simulink subsystem "anode_subsystem_basic_hctrl"  (R2023a)
settings: Solver=VariableStepAuto  StartTime=0.0  StopTime=10.0  RelTol=1e-3
values from neighbouring files (symbols this model uses):
  densityHydrogen = 0.0899    [All_Properties.mat]    (also in Valve_Init.m; anode_subsystem_parameters.m)
  Kv_VL6112 = 0.8    [All_Properties.mat]    (also in anode_subsystem_parameters.m)
undefined symbols (not defined in the file or in its folder): init_Parameters, ts
libraries: simulink x2, eeGeneralControl x1, slpidlib x1
settings Model: Creator=stefan.notter  LastModifiedBy=stefan.notter

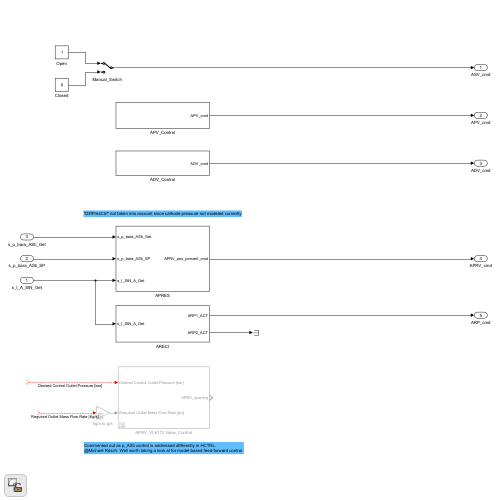
[thumbnail: Simulink's stored preview of the top-level diagram]
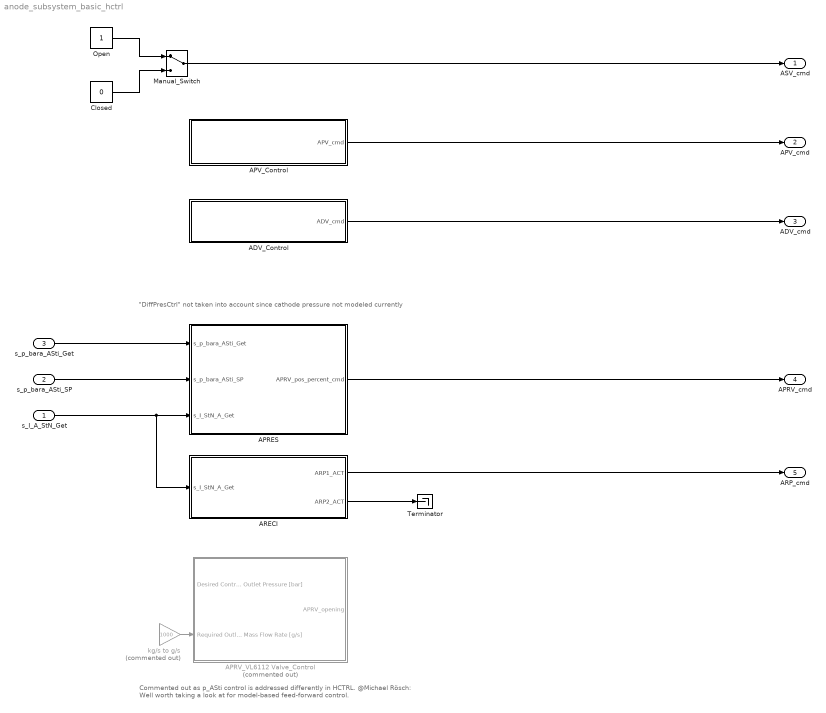
== system anode_subsystem_basic_hctrl ==
  note: Commented out as p_ASti control is addressed differently in HCTRL.
      | @Michael Rösch: Well worth taking a look at for model-based feed-forward control.
  note: "DiffPresCtrl" not taken into account since cathode pressure not modeled currently
  s_I_A_StN_Get : Inport
  s_p_bara_ASti_SP : Inport  Port=2
  s_p_bara_ASti_Get : Inport  Port=3
  ADV_Control : Subsystem
  APRES : Subsystem
  APRV_VL6112 Valve_Control : Subsystem  Commented=on
  APV_Control : Subsystem
  ARECI : Subsystem
  Closed : Constant  Value=0
  Manual_Switch : ManualSwitch
  Open : Constant
  Terminator : Terminator
  kg/s to g/s : Gain  Commented=on  Gain=1000
  ASV_cmd : Outport
  APV_cmd : Outport  Port=2
  ADV_cmd : Outport  Port=3
  APRV_cmd : Outport  Port=4
  ARP_cmd : Outport  Port=5
  wires:
  Closed/1 -> Manual_Switch/2
  Open/1 -> Manual_Switch/1
  Manual_Switch/1 -> ASV_cmd/1
  APV_Control/1(APV_cmd) -> APV_cmd/1
  ADV_Control/1(ADV_cmd) -> ADV_cmd/1
  kg/s to g/s/1 -> APRV_VL6112 Valve_Control/2(Required Outlet Mass Flow Rate [g/s])
  ? -> APRV_VL6112 Valve_Control/1(Desired Control Outlet Pressure [bar])  "Desired Control Outlet Pressure [bar]"
  ? -> kg/s to g/s/1  "Required Outlet Mass Flow Rate [Kg/s]"
  APRES/1(APRV_pos_percent_cmd) -> APRV_cmd/1
  ARECI/2(ARP2_ACT) -> Terminator/1
  ARECI/1(ARP1_ACT) -> ARP_cmd/1
  s_I_A_StN_Get/1 -> APRES/3(s_I_StN_A_Get), ARECI/1(s_I_StN_A_Get)
  s_p_bara_ASti_Get/1 -> APRES/1(s_p_bara_ASti_Get)
  s_p_bara_ASti_SP/1 -> APRES/2(s_p_bara_ASti_SP)

== system anode_subsystem_basic_hctrl/ADV_Control ==
  ADV orifice area : Gain  Gain=3.2e-6
  Periodic Default Drain Valve Signal : DiscretePulseGenerator  PulseType=Time based  Period=3  PulseWidth=5
  ADV_cmd : Outport
  wires:
  Periodic Default Drain Valve Signal/1 -> ADV orifice area/1
  ADV orifice area/1 -> ADV_cmd/1

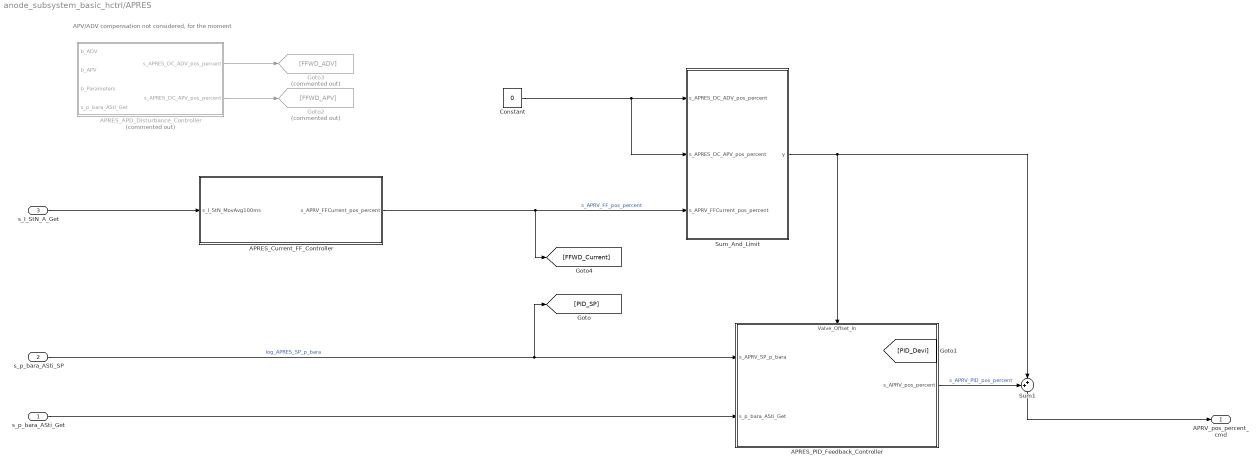
== system anode_subsystem_basic_hctrl/APRES ==
  note: APV/ADV compensation not considered, for the moment
  s_p_bara_ASti_Get : Inport
  s_p_bara_ASti_SP : Inport  Port=2
  s_I_StN_A_Get : Inport  Port=3
  APRES_APD_Disturbance_Controller : Subsystem  Commented=on
  APRES_Current_FF_Controller : Subsystem
  APRES_PID_Feedback_Controller : Subsystem
      settings: PortSchema="{\"entries\":[{\"content\":{\"sides\":[{\"content\":{\"connectorIds\":[\"In1\",\"In2\"]},\"type\":\"ConnectorPlacement.EquallySpacedRectSide\",\"uuid\":\"5897dec9-33fc-48cf-b321-aa2723f0279f\"},{\"content\":{\"connectorIds\":[\"Out1\"],\"side\":\"RIGHT\"},\"type\":\"ConnectorPlacement.EquallySpacedRectSide\",\"uuid\":\"dc72e443-0984-4518-a11e-1bbf1965bfdd\"},{\"content\":{\"connectorIds\":[\"In3\"],\"side\":\"TOP\"},\"type\":\"ConnectorPlacement.EquallySpacedRectSide\",\"uuid\":\"3eef5d8f-2798-4c48-9a57-b1498abce698\"}]},\"type\":\"ConnectorPlacement.EquallySpacedConnector\",\"uuid\":\"d7f9042a-4869-4dfe-bd3e-c21fb88551c7\"}],\"packageUris\":[\"http://schema.mathworks.com/mf0/Connector/R2020b\"],\"version\":\"1.0\"}"
  Constant : Constant  Value=0
  Goto2 : Goto  Commented=on  GotoTag=FFWD_APV
  Goto3 : Goto  Commented=on  GotoTag=FFWD_ADV
  Sum1 : Sum  Inputs=++|
  Sum_And_Limit : Subsystem
  APRV_pos_percent_cmd : Outport  PortDimensions=1
  wires:
  s_p_bara_ASti_Get/1 -> APRES_PID_Feedback_Controller/2(s_p_bara_ASti_Get)
  APRES_Current_FF_Controller/1(s_APRV_FFCurrent_pos_percent) -> Sum_And_Limit/3(s_APRV_FFCurrent_pos_percent), [FFWD_Current]  "s_APRV_FF_pos_percent"
  APRES_APD_Disturbance_Controller/1(s_APRES_DC_ADV_pos_percent) -> Goto3/1
  s_p_bara_ASti_SP/1 -> APRES_PID_Feedback_Controller/1(s_APRV_SP_p_bara), [PID_SP]  "log_APRES_SP_p_bara"
  APRES_APD_Disturbance_Controller/2(s_APRES_DC_APV_pos_percent) -> Goto2/1
  Sum_And_Limit/1(y) -> Sum1/2, APRES_PID_Feedback_Controller/3(Valve_Offset_In)
  Constant/1 -> Sum_And_Limit/1(s_APRES_DC_ADV_pos_percent), Sum_And_Limit/2(s_APRES_DC_APV_pos_percent)
  Sum1/1 -> APRV_pos_percent_cmd/1
  s_I_StN_A_Get/1 -> APRES_Current_FF_Controller/1(s_I_StN_MovAvg100ms)
  APRES_PID_Feedback_Controller/1(s_APRV_pos_percent) -> Sum1/1  "s_APRV_PID_pos_percent"

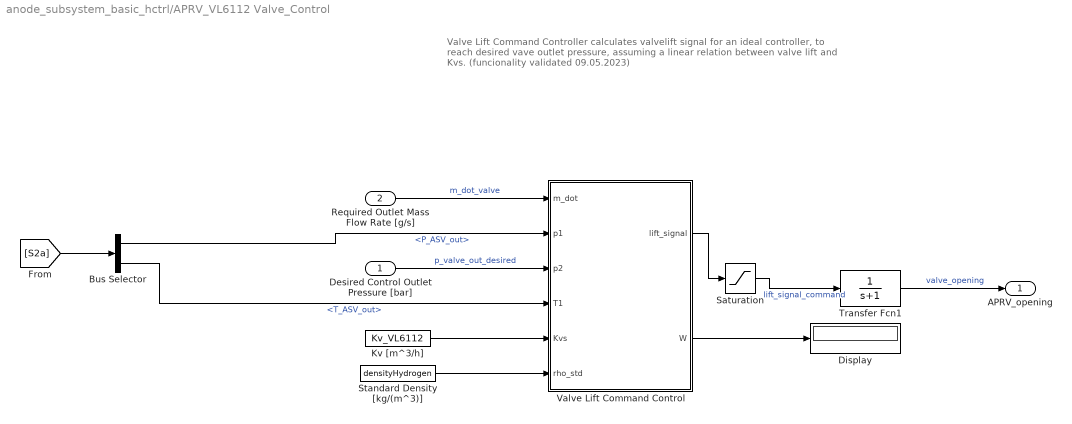
== system anode_subsystem_basic_hctrl/APRV_VL6112 Valve_Control ==
  note: Valve Lift Command Controller calculates valvelift signal for an
      | ideal controller, to reach desired vave outlet pressure, assuming
      | a linear relation between valve lift and Kvs.
      | (funcionality validated 09.05.2023)
  Desired Control Outlet Pressure [bar] : Inport
  Required Outlet Mass Flow Rate [g/s] : Inport  Port=2
  Bus Selector : BusSelector  OutputSignals=P_ASV_out,T_ASV_out
  Display : Display
  Kv [m^3/h] : Constant  Value=Kv_VL6112
  Saturation : Saturate  UpperLimit=1  LowerLimit=0
  Standard Density [kg/(m^3)] : Constant  Value=densityHydrogen
  Transfer Fcn1 : TransferFcn  Denominator=[1 1]
  Valve Lift Command Control : MATLAB Function  TreatAsAtomicUnit=on
  APRV_opening : Outport
  wires:
  [S2a] -> Bus Selector/1
  Saturation/1 -> Transfer Fcn1/1  "lift_signal_command"
  Desired Control Outlet Pressure [bar]/1 -> Valve Lift Command Control/3(p2)  "p_valve_out_desired"
  Bus Selector/2 -> Valve Lift Command Control/4(T1)  "<T_ASV_out>"
  Valve Lift Command Control/1(lift_signal) -> Saturation/1
  Standard Density [kg/(m^3)]/1 -> Valve Lift Command Control/6(rho_std)
  Kv [m^3/h]/1 -> Valve Lift Command Control/5(Kvs)
  Transfer Fcn1/1 -> APRV_opening/1  "valve_opening"
  Bus Selector/1 -> Valve Lift Command Control/2(p1)  "<P_ASV_out>"
  Valve Lift Command Control/2(W) -> Display/1
  Required Outlet Mass Flow Rate [g/s]/1 -> Valve Lift Command Control/1(m_dot)  "m_dot_valve"

== system anode_subsystem_basic_hctrl/APV_Control ==
  APV orifice area : Gain  Gain=3.2e-6
  Periodic Default Purge Signal : DiscretePulseGenerator  PulseType=Time based  Period=3  PulseWidth=5
  APV_cmd : Outport
  wires:
  APV orifice area/1 -> APV_cmd/1
  Periodic Default Purge Signal/1 -> APV orifice area/1

== system anode_subsystem_basic_hctrl/ARECI ==
  s_I_StN_A_Get : Inport
  LUT : Subsystem
  ARP1_ACT : Outport
  ARP2_ACT : Outport  Port=2
  wires:
  s_I_StN_A_Get/1 -> LUT/1(s_I_A_StN_Get)
  LUT/1(s_ARECI_SP_omega_rpm) -> ARP1_ACT/1, ARP2_ACT/1

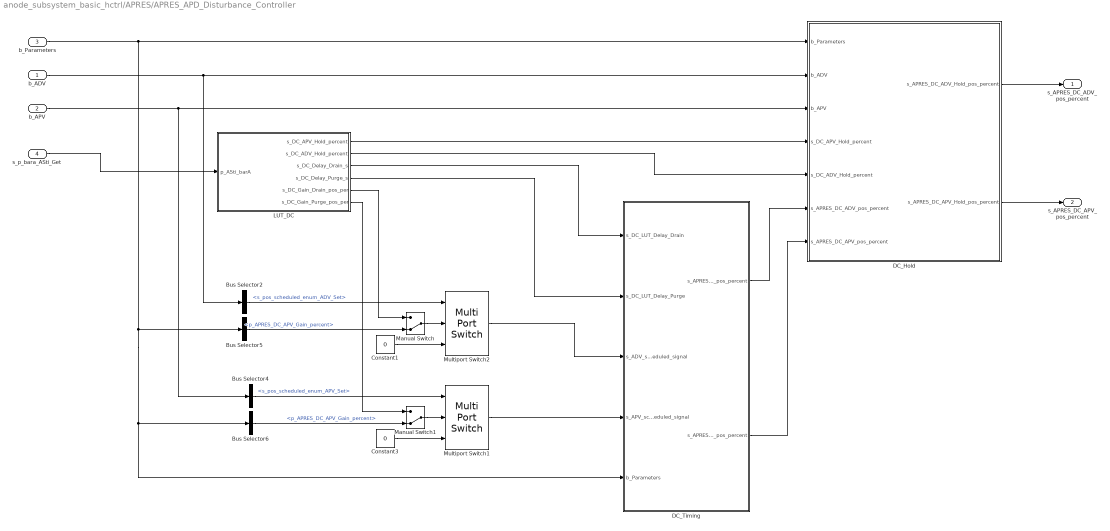
== system anode_subsystem_basic_hctrl/APRES/APRES_APD_Disturbance_Controller ==
  b_ADV : Inport  OutDataTypeStr=Bus: ADV
  b_APV : Inport  Port=2  OutDataTypeStr=Bus: APV
  b_Parameters : Inport  Port=3  OutDataTypeStr=Bus: Parameters
  s_p_bara_ASti_Get : Inport  Port=4
  Bus Selector2 : BusSelector  OutputSignals=s_pos_scheduled_enum_ADV_Set
  Bus Selector4 : BusSelector  OutputSignals=s_pos_scheduled_enum_APV_Set
  Bus Selector5 : BusSelector  OutputSignals=b_AN_Parameters.b_APRES_Parameters.p_APRES_DC_APV_Gain_percent
  Bus Selector6 : BusSelector  OutputSignals=b_AN_Parameters.b_APRES_Parameters.p_APRES_DC_APV_Gain_percent
  Constant1 : Constant  Value=0  OutDataTypeStr=single
  Constant3 : Constant  Value=0  OutDataTypeStr=single
  DC_Hold : Subsystem
  DC_Timing : Subsystem
  LUT_DC : Subsystem
  Manual Switch : ManualSwitch  CurrentSetting=0
  Manual Switch1 : ManualSwitch  CurrentSetting=0
  Multiport Switch1 : MultiPortSwitch  DataPortOrder=Specify indices  DataPortIndices={DVLV_STATE.Open, DVLV_STATE.Closed}  SaturateOnIntegerOverflow=off  InputSameDT=off
  Multiport Switch2 : MultiPortSwitch  DataPortOrder=Specify indices  DataPortIndices={DVLV_STATE.Open, DVLV_STATE.Closed}  SaturateOnIntegerOverflow=off  InputSameDT=off
  s_APRES_DC_ADV_pos_percent : Outport
  s_APRES_DC_APV_pos_percent : Outport  Port=2
  wires:
  s_p_bara_ASti_Get/1 -> LUT_DC/1(p_ASti_barA)
  b_ADV/1 -> DC_Hold/2(b_ADV), Bus Selector2/1
  Constant1/1 -> Multiport Switch2/3
  Bus Selector4/1 -> Multiport Switch1/1  "<s_pos_scheduled_enum_APV_Set>"
  Multiport Switch2/1 -> DC_Timing/3(s_ADV_scheduled_signal)
  DC_Timing/1(s_APRES_DC_ADV_pos_percent) -> DC_Hold/6(s_APRES_DC_ADV_pos_percent)
  Multiport Switch1/1 -> DC_Timing/4(s_APV_scheduled_signal)
  Bus Selector2/1 -> Multiport Switch2/1  "<s_pos_scheduled_enum_ADV_Set>"
  Constant3/1 -> Multiport Switch1/3
  b_Parameters/1 -> DC_Hold/1(b_Parameters), Bus Selector5/1, Bus Selector6/1, DC_Timing/5(b_Parameters)
  DC_Hold/1(s_APRES_DC_ADV_Hold_pos_percent) -> s_APRES_DC_ADV_pos_percent/1
  DC_Hold/2(s_APRES_DC_APV_Hold_pos_percent) -> s_APRES_DC_APV_pos_percent/1
  Manual Switch1/1 -> Multiport Switch1/2
  LUT_DC/2(s_DC_ADV_Hold_percent) -> DC_Hold/5(s_DC_ADV_Hold_percent)
  DC_Timing/2(s_APRES_DC_APV_pos_percent) -> DC_Hold/7(s_APRES_DC_APV_pos_percent)
  Bus Selector5/1 -> Manual Switch/2  "<p_APRES_DC_APV_Gain_percent>"
  Manual Switch/1 -> Multiport Switch2/2
  LUT_DC/1(s_DC_APV_Hold_percent) -> DC_Hold/4(s_DC_APV_Hold_percent)
  LUT_DC/6(s_DC_Gain_Purge_pos_per) -> Manual Switch1/1
  LUT_DC/5(s_DC_Gain_Drain_pos_per) -> Manual Switch/1
  b_APV/1 -> DC_Hold/3(b_APV), Bus Selector4/1
  Bus Selector6/1 -> Manual Switch1/2  "<p_APRES_DC_APV_Gain_percent>"
  LUT_DC/4(s_DC_Delay_Purge_s) -> DC_Timing/2(s_DC_LUT_Delay_Purge)
  LUT_DC/3(s_DC_Delay_Drain_s) -> DC_Timing/1(s_DC_LUT_Delay_Drain)

== system anode_subsystem_basic_hctrl/APRES/APRES_Current_FF_Controller ==
  s_I_StN_MovAvg100ms : Inport
  Constant : Constant  Value=0  OutDataTypeStr=single
  LUT_APRV_FF_Current : Lookup_n-D  NumberOfTableDimensions=1  BreakpointsForDimension1="[0    10  20  30  40  50      75  100   150     200     250     300     350     400]"  Table="[35   36  37  39  42  44.9    50.3  50.7 \t53.5    56.9    60.4    63.4    66.1    66.1]"  ExtrapMethod=Clip  UseLastTableValue=on  InternalRulePriority=Speed  RndMeth=Simplest
  Manual Switch : ManualSwitch  CurrentSetting=0
  Moving Average (Variable Frequency) : eeGeneralControl/Moving Average (Variable Frequency)  VariantControl=Variant1  LabelModeActiveChoice=Discrete  f0=100  fmin=1  x0=0  BufferSize=8192  Ts=-1
      settings: LibrarySourceBlock=|
      | ee_sl_lib/General Control/Moving Average
      | (Variable Frequency)
  p_APRES_FFCurr_FilterFreq_Hz : Constant  Value=100
  s_APRV_FFCurrent_pos_percent : Outport
  wires:
  Manual Switch/1 -> s_APRV_FFCurrent_pos_percent/1
  LUT_APRV_FF_Current/1 -> Manual Switch/2
  p_APRES_FFCurr_FilterFreq_Hz/1 -> Moving Average (Variable Frequency)/1
  s_I_StN_MovAvg100ms/1 -> Moving Average (Variable Frequency)/2
  Moving Average (Variable Frequency)/1 -> LUT_APRV_FF_Current/1
  Constant/1 -> Manual Switch/1

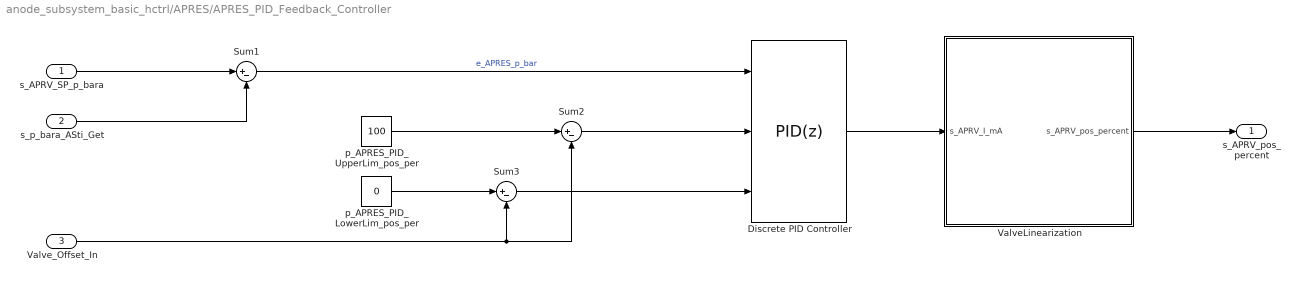
== system anode_subsystem_basic_hctrl/APRES/APRES_PID_Feedback_Controller ==
  s_APRV_SP_p_bara : Inport
  s_p_bara_ASti_Get : Inport  Port=2
  Valve_Offset_In : Inport  Port=3
  Discrete PID Controller : slpidlib/PID Controller  Controller=PID  Form=Parallel  TimeDomain=Discrete-time  UseExternalTs=off  SampleTime=-1  IntegratorMethod=Trapezoidal  FilterMethod=Trapezoidal  ControllerParametersSource=internal  P=90  I=40  UseKiTs=off  D=0  N=100  UseFilter=off  TunerSelectOption=Transfer Function Based (PID Tuner App)  InitialConditionSource=internal  InitialConditionForIntegrator=0  InitialConditionForFilter=0  DifferentiatorICPrevScaledInput=0  ExternalReset=none  TrackingMode=off  Kt=1  LimitOutput=on  SatLimitsSource=external  UpperSaturationLimit=inf  LowerSaturationLimit=-inf  LinearizeAsGain=off  AntiWindupMode=clamping  Kb=1  LimitIntegrator=on  UpperIntegratorSaturationLimit=10000  LowerIntegratorSaturationLimit=-10000  POutMin=[]  POutMax=[]  IOutMin=[]  IOutMax=[]  DOutMin=[]  DOutMax=[]  NOutMin=[]  NOutMax=[]  SumOutMin=[]  SumOutMax=[]  SaturationOutMin=[]  SaturationOutMax=[]  PParamMin=[]  PParamMax=[]  IParamMin=[]  IParamMax=[]  DParamMin=[]  DParamMax=[]  NParamMin=[]  NParamMax=[]  KbParamMin=[]  KbParamMax=[]  KtParamMin=[]  KtParamMax=[]  KbOutMin=[]  KbOutMax=[]  KtOutMin=[]  KtOutMax=[]  IntegratorOutMin=[]  IntegratorOutMax=[]  FilterOutMin=[]  FilterOutMax=[]  SumI1OutMin=[]  SumI1OutMax=[]  SumI2OutMin=[]  SumI2OutMax=[]  SumI3OutMin=[]  SumI3OutMax=[]  SumI4OutMin=[]  SumI4OutMax=[]  SumDOutMin=[]  SumDOutMax=[]  DifferentiatorOutMin=[]  DifferentiatorOutMax=[]  FilterDiffOutCoefMin=[]  FilterDiffOutCoefMax=[]  ReciprocalOutMin=[]  ReciprocalOutMax=[]  SumDenOutMin=[]  SumDenOutMax=[]  SumNumOutMin=[]  SumNumOutMax=[]  DivideOutMin=[]  DivideOutMax=[]  UdiffTsProdOutMin=[]  UdiffTsProdOutMax=[]  NTsProdOutMin=[]  NTsProdOutMax=[]  UintegralTsProdOutMin=[]  UintegralTsProdOutMax=[]  UngainTsProdOutMin=[]  UngainTsProdOutMax=[]  ClampingZeroOutDataTypeStr=Inherit: Inherit via back propagation  ClampingZeroOutMin=[]  ClampingZeroOutMax=[]  FilterDenConstantOutDataTypeStr=Inherit: Inherit via back propagation  FilterDenConstantOutMin=[]  FilterDenConstantOutMax=[]  PCopyOutDataTypeStr=Inherit: Inherit via back propagation  PCopyOutMin=[]  PCopyOutMax=[]  NCopyOutDataTypeStr=Inherit: Inherit via back propagation  NCopyOutMin=[]  NCopyOutMax=[]  IntegratorContinuousStateAttributes=''  IntegratorStateMustResolveToSignalObject=off  IntegratorRTWStateStorageClass=Auto  FilterContinuousStateAttributes=''  FilterStateMustResolveToSignalObject=off  FilterRTWStateStorageClass=Auto  ParallelPVariant=InternalParameters  IdealPVariant=Disabled  IVariant=InternalParameters  DVariant=InternalParameters  IntegratorVariant=Discrete  SatVariant=External  AWVariant=DiscClampingParallel  PCopyVariant=Disabled  TRVariant=Disabled  FdbkBlocksVariant=Feedback  IdealPFdbkVariant=Passthrough  SatFdbkVariant=Passthrough  DerivativeFilterVariant=Differentiator  NVariant=Passthrough  NCopyVariant=Disabled_SignalSpec  FilterICVariant=InternalICsDifferentiator  IntegratorICVariant=InternalICs  ExternalResetVariant=Disabled  TRSumVariant=Passthrough  SumFdbkVariant=Enabled  SumVariant=Sum_PID  TsampFilterVariant=InternalTs  TsampNgainVariant=Passthrough  TsampIntegralVariant=Disabled_SignalSpec  ExternalSaturationOutDataTypeStr=Inherit: Same as second input
      settings: LibrarySourceBlock=simulink/Discrete/Discrete PID Controller
  Sum1 : Sum  Inputs=|+-
  Sum2 : Sum  Inputs=|+-
  Sum3 : Sum  Inputs=|+-
  ValveLinearization : Subsystem
  p_APRES_PID_LowerLim_pos_per : Constant  Value=0
  p_APRES_PID_UpperLim_pos_per : Constant  Value=100
  s_APRV_pos_percent : Outport
  wires:
  Sum2/1 -> Discrete PID Controller/2
  ValveLinearization/1(s_APRV_pos_percent) -> s_APRV_pos_percent/1
  Sum1/1 -> Discrete PID Controller/1  "e_APRES_p_bar"
  s_APRV_SP_p_bara/1 -> Sum1/1
  Discrete PID Controller/1 -> ValveLinearization/1(s_APRV_I_mA)
  s_p_bara_ASti_Get/1 -> Sum1/2
  Sum3/1 -> Discrete PID Controller/3
  Valve_Offset_In/1 -> Sum3/2, Sum2/2
  p_APRES_PID_LowerLim_pos_per/1 -> Sum3/1
  p_APRES_PID_UpperLim_pos_per/1 -> Sum2/1

== system anode_subsystem_basic_hctrl/APRES/Sum_And_Limit ==
  s_APRES_DC_ADV_pos_percent : Inport
  s_APRES_DC_APV_pos_percent : Inport  Port=2
  s_APRV_FFCurrent_pos_percent : Inport  Port=3
  Saturation Dynamic : simulink/Discontinuities/Saturation Dynamic  OutMin=[]  OutMax=[]  OutDataTypeStr=Inherit: Same as second input  OutDataType=fixdt(1, 16)  OutScaling=2^-10  DoSatur=off
  Sum1 : Sum  Inputs=+++
  p_APRES_PID_LowerLim_pos_per : Constant  Value=0
  p_APRES_PID_UpperLim_pos_per : Constant  Value=100
  y : Outport
  wires:
  Sum1/1 -> Saturation Dynamic/2
  s_APRV_FFCurrent_pos_percent/1 -> Sum1/3
  p_APRES_PID_UpperLim_pos_per/1 -> Saturation Dynamic/1
  s_APRES_DC_APV_pos_percent/1 -> Sum1/2
  s_APRES_DC_ADV_pos_percent/1 -> Sum1/1
  p_APRES_PID_LowerLim_pos_per/1 -> Saturation Dynamic/3
  Saturation Dynamic/1 -> y/1

== system anode_subsystem_basic_hctrl/ARECI/LUT ==
  note: commented out here since current dynamics are not modeled, so far
  s_I_A_StN_Get : Inport
  Delay_Or_Precontrol_ARECI : Subsystem  Commented=on
  LUT_ARECI_FF_Current : Lookup_n-D  NumberOfTableDimensions=1  BreakpointsForDimension1="[0      50      100     150     200     250     300     350     400     425     450     475     500]"  Table="[2500   2500    2500    3000    4500    5000    5000    5200    5200    5200    5200    5200    5200]"  ExtrapMethod=Clip  UseLastTableValue=on  InternalRulePriority=Speed  RndMeth=Simplest
  s_ARECI_SP_omega_rpm : Outport  PortDimensions=1
  wires:
  s_I_A_StN_Get/1 -> LUT_ARECI_FF_Current/1
  LUT_ARECI_FF_Current/1 -> s_ARECI_SP_omega_rpm/1

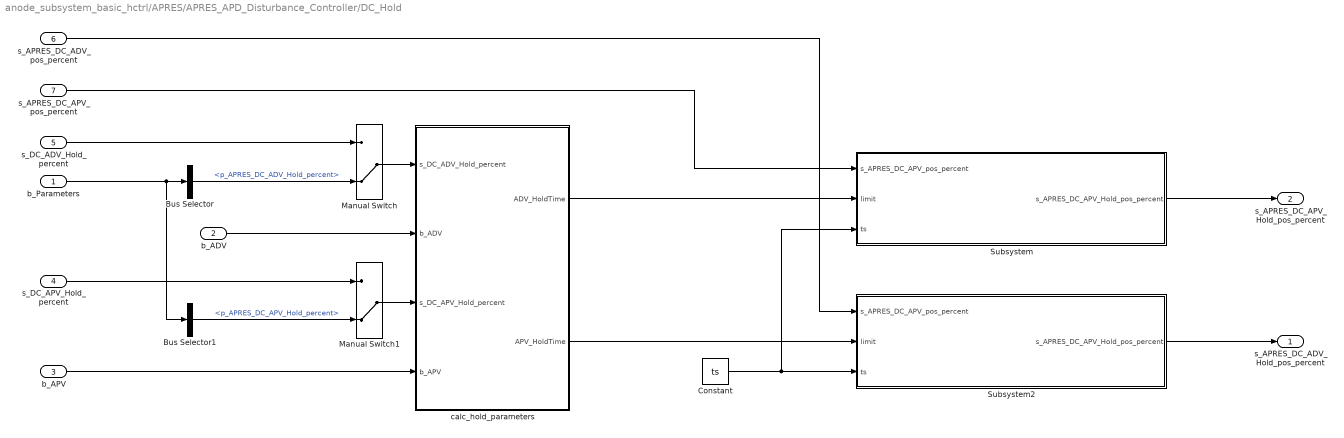
== system anode_subsystem_basic_hctrl/APRES/APRES_APD_Disturbance_Controller/DC_Hold ==
  b_Parameters : Inport  OutDataTypeStr=Bus: Parameters
  b_ADV : Inport  Port=2
  b_APV : Inport  Port=3
  s_DC_APV_Hold_percent : Inport  Port=4
  s_DC_ADV_Hold_percent : Inport  Port=5
  s_APRES_DC_ADV_pos_percent : Inport  Port=6
  s_APRES_DC_APV_pos_percent : Inport  Port=7
  Bus Selector : BusSelector  OutputSignals=b_AN_Parameters.b_APRES_Parameters.p_APRES_DC_ADV_Hold_percent
  Bus Selector1 : BusSelector  OutputSignals=b_AN_Parameters.b_APRES_Parameters.p_APRES_DC_APV_Hold_percent
  Constant : Constant  Value=ts  OutDataTypeStr=single
  Manual Switch : ManualSwitch  CurrentSetting=0
  Manual Switch1 : ManualSwitch  CurrentSetting=0
  Subsystem : Subsystem
  Subsystem2 : Subsystem
  calc_hold_parameters : Subsystem
  s_APRES_DC_ADV_Hold_pos_percent : Outport
  s_APRES_DC_APV_Hold_pos_percent : Outport  Port=2
  wires:
  Constant/1 -> Subsystem2/3(ts), Subsystem/3(ts)
  Subsystem2/1(s_APRES_DC_APV_Hold_pos_percent) -> s_APRES_DC_ADV_Hold_pos_percent/1
  Subsystem/1(s_APRES_DC_APV_Hold_pos_percent) -> s_APRES_DC_APV_Hold_pos_percent/1
  Bus Selector1/1 -> Manual Switch1/2  "<p_APRES_DC_APV_Hold_percent>"
  Bus Selector/1 -> Manual Switch/2  "<p_APRES_DC_ADV_Hold_percent>"
  Manual Switch1/1 -> calc_hold_parameters/3(s_DC_APV_Hold_percent)
  Manual Switch/1 -> calc_hold_parameters/1(s_DC_ADV_Hold_percent)
  b_Parameters/1 -> Bus Selector/1, Bus Selector1/1
  calc_hold_parameters/2(APV_HoldTime) -> Subsystem2/2(limit)
  calc_hold_parameters/1(ADV_HoldTime) -> Subsystem/2(limit)
  b_APV/1 -> calc_hold_parameters/4(b_APV)
  s_DC_APV_Hold_percent/1 -> Manual Switch1/1
  b_ADV/1 -> calc_hold_parameters/2(b_ADV)
  s_DC_ADV_Hold_percent/1 -> Manual Switch/1
  s_APRES_DC_ADV_pos_percent/1 -> Subsystem2/1(s_APRES_DC_APV_pos_percent)
  s_APRES_DC_APV_pos_percent/1 -> Subsystem/1(s_APRES_DC_APV_pos_percent)

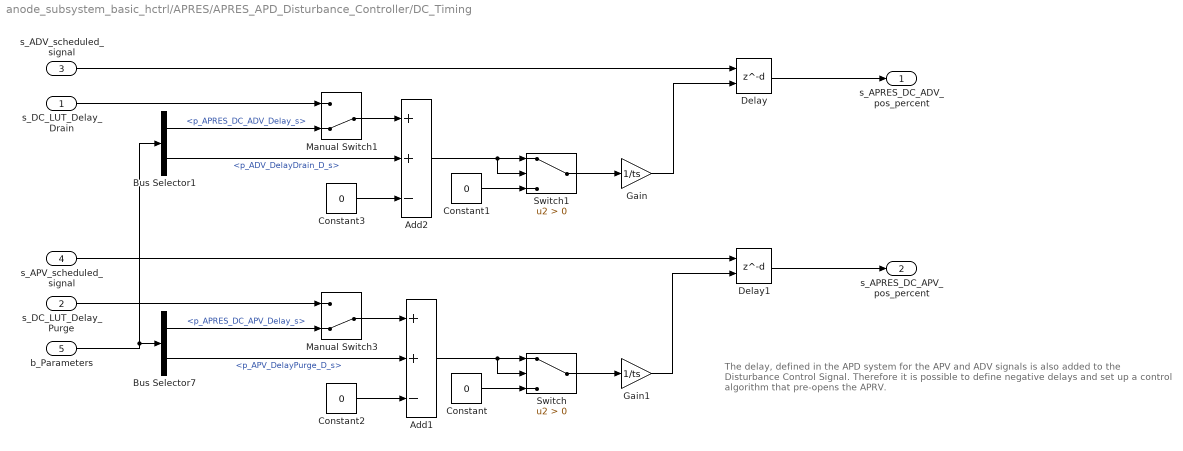
== system anode_subsystem_basic_hctrl/APRES/APRES_APD_Disturbance_Controller/DC_Timing ==
  note: The delay, defined in the APD system for the APV and ADV signals is also added to the Disturbance Control Signal. Therefore it is possible to define negative delays and set up a control algorithm that pre-opens the APRV.
  s_DC_LUT_Delay_Drain : Inport
  s_DC_LUT_Delay_Purge : Inport  Port=2
  s_ADV_scheduled_signal : Inport  Port=3
  s_APV_scheduled_signal : Inport  Port=4
  b_Parameters : Inport  Port=5  OutDataTypeStr=Bus: Parameters
  Add1 : Sum  Inputs=++-
  Add2 : Sum  Inputs=++-
  Bus Selector1 : BusSelector  OutputSignals=b_AN_Parameters.b_APRES_Parameters.p_APRES_DC_ADV_Delay_s,b_AN_Parameters.b_APD_Parameters.p_ADV_DelayDrain_D_s
  Bus Selector7 : BusSelector  OutputSignals=b_AN_Parameters.b_APRES_Parameters.p_APRES_DC_APV_Delay_s,b_AN_Parameters.b_APD_Parameters.p_APV_DelayPurge_D_s
  Constant{,1..3} (4 alike) : Constant  Value=0  OutDataTypeStr=single
  Delay : Delay  DelayLengthSource=Input port  DelayLength=init_Parameters.b_AN_Parameters.b_APRES_Parameters.p_APRES_APV_FeedForwardDelay_s/ts
      settings: InputPortMap=u0,p1
  Delay1 : Delay  DelayLengthSource=Input port  DelayLength=init_Parameters.b_AN_Parameters.b_APRES_Parameters.p_APRES_ADV_FeedForwardDelay_s/ts
      settings: InputPortMap=u0,p1
  Gain : Gain  Gain=1/ts
  Gain1 : Gain  Gain=1/ts
  Manual Switch1 : ManualSwitch  CurrentSetting=0
  Manual Switch3 : ManualSwitch  CurrentSetting=0
  Switch : Switch  Criteria=u2 > Threshold  SaturateOnIntegerOverflow=off  InputSameDT=off
  Switch1 : Switch  Criteria=u2 > Threshold  SaturateOnIntegerOverflow=off  InputSameDT=off
  s_APRES_DC_ADV_pos_percent : Outport
  s_APRES_DC_APV_pos_percent : Outport  Port=2
  wires:
  Constant3/1 -> Add2/3
  Constant2/1 -> Add1/3
  Switch1/1 -> Gain/1
  Add2/1 -> Switch1/1, Switch1/2
  Constant1/1 -> Switch1/3
  Constant/1 -> Switch/3
  Add1/1 -> Switch/1, Switch/2
  Manual Switch3/1 -> Add1/1
  Switch/1 -> Gain1/1
  Bus Selector7/2 -> Add1/2  "<p_APV_DelayPurge_D_s>"
  Bus Selector1/2 -> Add2/2  "<p_ADV_DelayDrain_D_s>"
  Bus Selector1/1 -> Manual Switch1/2  "<p_APRES_DC_ADV_Delay_s>"
  s_DC_LUT_Delay_Drain/1 -> Manual Switch1/1
  s_DC_LUT_Delay_Purge/1 -> Manual Switch3/1
  s_ADV_scheduled_signal/1 -> Delay/1
  b_Parameters/1 -> Bus Selector7/1, Bus Selector1/1
  Manual Switch1/1 -> Add2/1
  Gain1/1 -> Delay1/2
  Delay1/1 -> s_APRES_DC_APV_pos_percent/1
  Gain/1 -> Delay/2
  s_APV_scheduled_signal/1 -> Delay1/1
  Bus Selector7/1 -> Manual Switch3/2  "<p_APRES_DC_APV_Delay_s>"
  Delay/1 -> s_APRES_DC_ADV_pos_percent/1

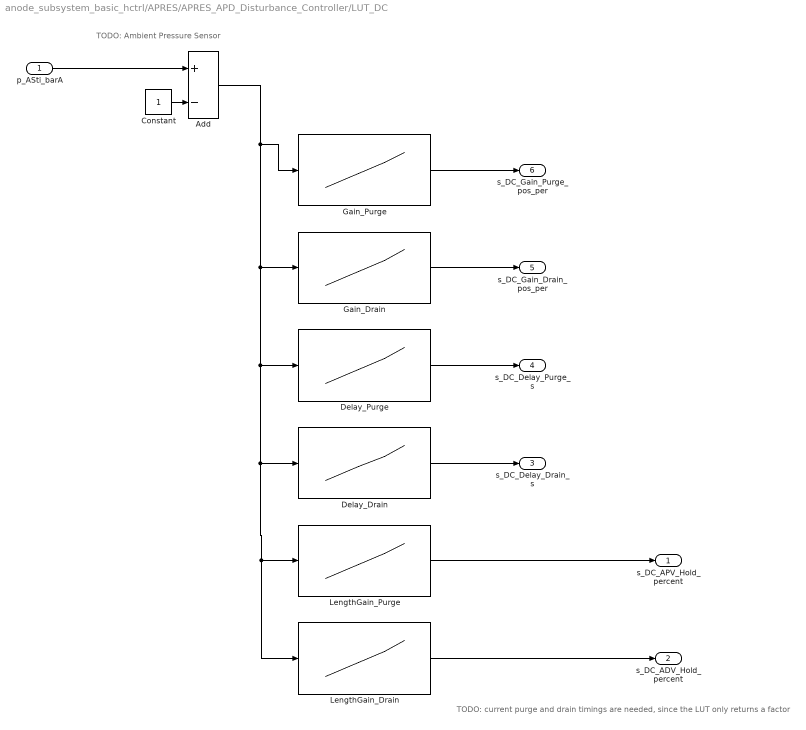
== system anode_subsystem_basic_hctrl/APRES/APRES_APD_Disturbance_Controller/LUT_DC ==
  note: TODO: current purge and drain timings are needed, since the LUT only returns a factor
  note: TODO: Ambient Pressure Sensor
  p_ASti_barA : Inport
  Add : Sum  Inputs=+-
  Constant : Constant  OutDataTypeStr=single
  Delay_Drain : Lookup_n-D  NumberOfTableDimensions=1  BreakpointsForDimension1=[0, 0.05, 0.1, 0.15, 0.2, 0.25, 0.3, 0.4, 0.5, 0.6, 0.7, 0.8, 1, 1.1]  Table=[0.01, 0.01, 0.01, 0.01, 0.01, 0.01, 0.01, 0.01, 0.01, 0.01, 0.01, 0.01, 0.01, 0.01]  ExtrapMethod=Clip  UseLastTableValue=on  InternalRulePriority=Speed  RndMeth=Simplest
  Delay_Purge : Lookup_n-D  NumberOfTableDimensions=1  BreakpointsForDimension1=[0, 0.05, 0.1, 0.15, 0.2, 0.25, 0.3, 0.4, 0.5, 0.6, 0.7, 0.8, 1, 1.1]  Table=[0.01, 0.01, 0.01, 0.01, 0.01, 0.01, 0.01, 0.01, 0.01, 0.01, 0.01, 0.01, 0.01, 0.01]  ExtrapMethod=Clip  UseLastTableValue=on  InternalRulePriority=Speed  RndMeth=Simplest
  Gain_Drain : Lookup_n-D  NumberOfTableDimensions=1  BreakpointsForDimension1=[0, 0.05, 0.1, 0.15, 0.2, 0.25, 0.3, 0.4, 0.5, 0.6, 0.7, 0.8, 1, 1.1]  Table=[12, 12, 12, 12, 12, 12, 12, 12, 12, 12, 12, 12, 12, 12]  ExtrapMethod=Clip  UseLastTableValue=on  InternalRulePriority=Speed  RndMeth=Simplest
  Gain_Purge : Lookup_n-D  NumberOfTableDimensions=1  BreakpointsForDimension1=[0, 0.05, 0.1, 0.15, 0.2, 0.25, 0.3, 0.4, 0.5, 0.6, 0.7, 0.8, 1, 1.1]  Table=[12, 12, 12, 12, 12, 12, 12, 12, 12, 12, 12, 12, 12, 12]  ExtrapMethod=Clip  UseLastTableValue=on  InternalRulePriority=Speed  RndMeth=Simplest
  LengthGain_Drain : Lookup_n-D  NumberOfTableDimensions=1  BreakpointsForDimension1=[0, 0.05, 0.1, 0.15, 0.2, 0.25, 0.3, 0.4, 0.5, 0.6, 0.7, 0.8, 1, 1.1]  Table=[100, 100, 100, 100, 100, 100, 100, 100, 100, 100, 100, 100, 100, 100]  ExtrapMethod=Clip  UseLastTableValue=on  InternalRulePriority=Speed  RndMeth=Simplest
  LengthGain_Purge : Lookup_n-D  NumberOfTableDimensions=1  BreakpointsForDimension1=[0, 0.05, 0.1, 0.15, 0.2, 0.25, 0.3, 0.4, 0.5, 0.6, 0.7, 0.8, 1, 1.1]  Table=[100, 100, 100, 100, 100, 100, 100, 100, 100, 100, 100, 100, 100, 100]  ExtrapMethod=Clip  UseLastTableValue=on  InternalRulePriority=Speed  RndMeth=Simplest
  s_DC_APV_Hold_percent : Outport
  s_DC_ADV_Hold_percent : Outport  Port=2
  s_DC_Delay_Drain_s : Outport  Port=3
  s_DC_Delay_Purge_s : Outport  Port=4
  s_DC_Gain_Drain_pos_per : Outport  Port=5
  s_DC_Gain_Purge_pos_per : Outport  Port=6
  wires:
  Gain_Purge/1 -> s_DC_Gain_Purge_pos_per/1
  Gain_Drain/1 -> s_DC_Gain_Drain_pos_per/1
  p_ASti_barA/1 -> Add/1
  Constant/1 -> Add/2
  Add/1 -> LengthGain_Drain/1, LengthGain_Purge/1, Delay_Drain/1, Delay_Purge/1, Gain_Drain/1, Gain_Purge/1
  Delay_Purge/1 -> s_DC_Delay_Purge_s/1
  Delay_Drain/1 -> s_DC_Delay_Drain_s/1
  LengthGain_Purge/1 -> s_DC_APV_Hold_percent/1
  LengthGain_Drain/1 -> s_DC_ADV_Hold_percent/1

== system anode_subsystem_basic_hctrl/APRES/APRES_PID_Feedback_Controller/ValveLinearization ==
  s_APRV_I_mA : Inport
  Bus Selector1 : BusSelector  Commented=on  OutputSignals=b_AN_Parameters.b_APRES_Parameters.p_APRV_ValveCurrnLUT_I_mA,b_AN_Parameters.b_APRES_Parameters.p_APRV_ValveCurrLUT_pos_per
  ValveCurrentLinearization : simulink/Lookup Tables/Lookup Table Dynamic  Commented=on  LookUpMeth=Interpolation-Use End Values  OutDataType=fixdt('double')  OutScaling=[]  OutputDataTypeScalingMode=Specify via dialog  OutDataTypeStr=double  DoSatur=off
  s_APRV_pos_percent : Outport
  wires:
  s_APRV_I_mA/1 -> s_APRV_pos_percent/1  "s_APRV_pos_percent"
  Bus Selector1/2 -> ValveCurrentLinearization/3  "<p_APRV_ValveCurrLUT_pos_per>"
  Bus Selector1/1 -> ValveCurrentLinearization/2  "<p_APRV_ValveCurrnLUT_I_mA>"

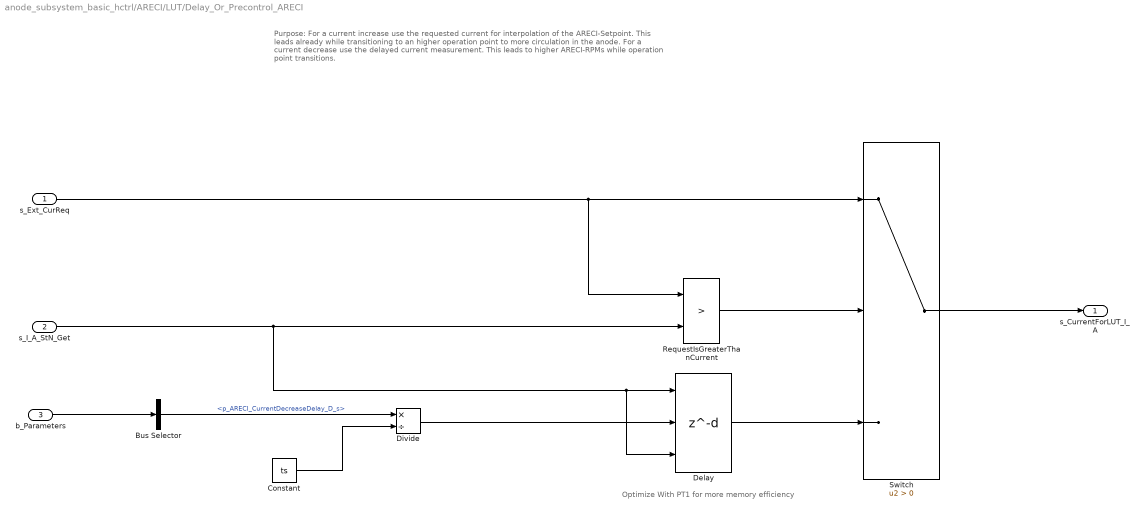
== system anode_subsystem_basic_hctrl/ARECI/LUT/Delay_Or_Precontrol_ARECI ==
  note: Optimize With PT1 for more memory efficiency
  note: Purpose: For a current increase use the requested current for interpolation of the ARECI-Setpoint. This leads already while transitioning to an higher operation point to more circulation in the anode.
      | For a current decrease use the delayed current measurement. This leads to higher ARECI-RPMs while operation point transitions.
  s_Ext_CurReq : Inport  BusOutputAsStruct=on
  s_I_A_StN_Get : Inport  Port=2
  b_Parameters : Inport  Port=3  OutDataTypeStr=Bus: Parameters
  Bus Selector : BusSelector  OutputSignals=b_AN_Parameters.b_ARECI_Parameters.p_ARECI_CurrentDecreaseDelay_D_s
  Constant : Constant  Value=ts  OutDataTypeStr=single
  Delay : Delay  DelayLengthSource=Input port  DelayLengthUpperLimit=1100  InitialConditionSource=Input port
      settings: InputPortMap=u0,p1,p4
  Divide : Product  Inputs=*/
  RequestIsGreaterThanCurrent : RelationalOperator  Operator=>  OutDataTypeStr=boolean  RndMeth=Simplest  InputSameDT=off
  Switch : Switch  Criteria=u2 > Threshold  SaturateOnIntegerOverflow=off  InputSameDT=off
  s_CurrentForLUT_I_A : Outport
  wires:
  s_Ext_CurReq/1 -> Switch/1, RequestIsGreaterThanCurrent/1
  Switch/1 -> s_CurrentForLUT_I_A/1
  Constant/1 -> Divide/2
  Bus Selector/1 -> Divide/1  "<p_ARECI_CurrentDecreaseDelay_D_s>"
  b_Parameters/1 -> Bus Selector/1
  Divide/1 -> Delay/2
  Delay/1 -> Switch/3
  RequestIsGreaterThanCurrent/1 -> Switch/2
  s_I_A_StN_Get/1 -> RequestIsGreaterThanCurrent/2, Delay/1, Delay/3

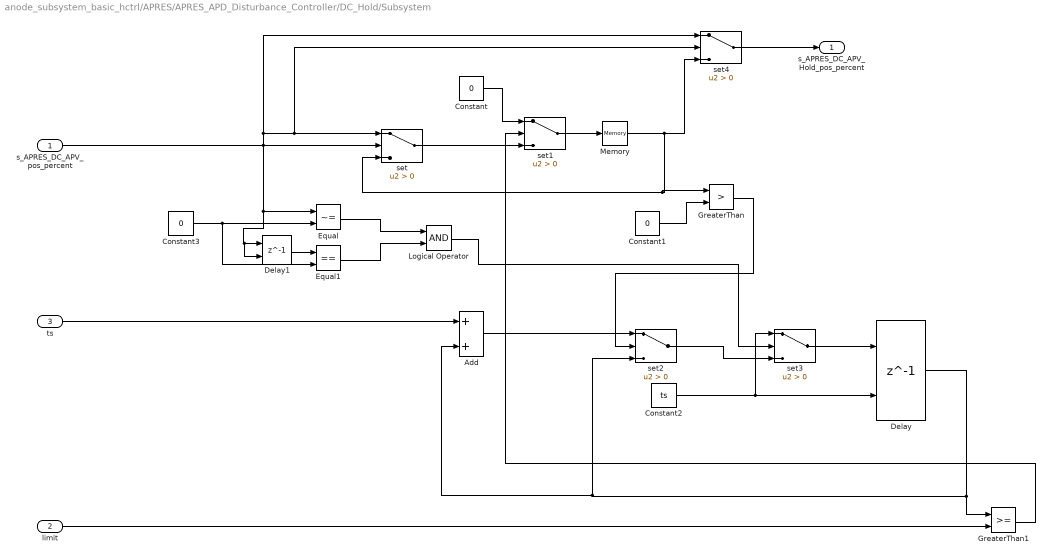
== system anode_subsystem_basic_hctrl/APRES/APRES_APD_Disturbance_Controller/DC_Hold/Subsystem ==
  s_APRES_DC_APV_pos_percent : Inport
  limit : Inport  Port=2
  ts : Inport  Port=3
  Add : Sum
  Constant : Constant  Value=0  OutDataTypeStr=single
  Constant1 : Constant  Value=0  OutDataTypeStr=single
  Constant2 : Constant  Value=ts  OutDataTypeStr=single
  Constant3 : Constant  Value=0  OutDataTypeStr=single
  Delay : Delay  DelayLength=1  InitialConditionSource=Input port
      settings: InputPortMap=u0,p4
  Delay1 : Delay  DelayLength=1  InitialConditionSource=Input port
      settings: InputPortMap=u0,p4
  Equal : RelationalOperator  Operator=~=  OutDataTypeStr=boolean  RndMeth=Simplest  InputSameDT=off
  Equal1 : RelationalOperator  Operator===  OutDataTypeStr=boolean  RndMeth=Simplest  InputSameDT=off
  GreaterThan : RelationalOperator  Operator=>  OutDataTypeStr=boolean  RndMeth=Simplest  InputSameDT=off
  GreaterThan1 : RelationalOperator  OutDataTypeStr=boolean  RndMeth=Simplest  InputSameDT=off
  Logical Operator : Logic  AllPortsSameDT=off  OutDataTypeStr=boolean
  Memory : Memory
  set{,1..4} (5 alike) : Switch  Criteria=u2 > Threshold  SaturateOnIntegerOverflow=off  InputSameDT=off
  s_APRES_DC_APV_Hold_pos_percent : Outport
  wires:
  Memory/1 -> GreaterThan/1, set/3, set4/3
  set/1 -> set1/3
  set1/1 -> Memory/1
  Constant/1 -> set1/1
  Constant1/1 -> GreaterThan/2
  Constant2/1 -> set3/1, Delay/2
  Add/1 -> set2/1
  Delay/1 -> GreaterThan1/1, set2/3, Add/2
  ts/1 -> Add/1
  limit/1 -> GreaterThan1/2
  GreaterThan1/1 -> set1/2
  GreaterThan/1 -> set2/2
  set2/1 -> set3/3
  Constant3/1 -> Equal/2, Equal1/2
  s_APRES_DC_APV_pos_percent/1 -> Delay1/2, Delay1/1, Equal/1, set4/1, set4/2, set/1, set/2
  Delay1/1 -> Equal1/1
  Equal/1 -> Logical Operator/1
  Equal1/1 -> Logical Operator/2
  Logical Operator/1 -> set3/2
  set3/1 -> Delay/1
  set4/1 -> s_APRES_DC_APV_Hold_pos_percent/1

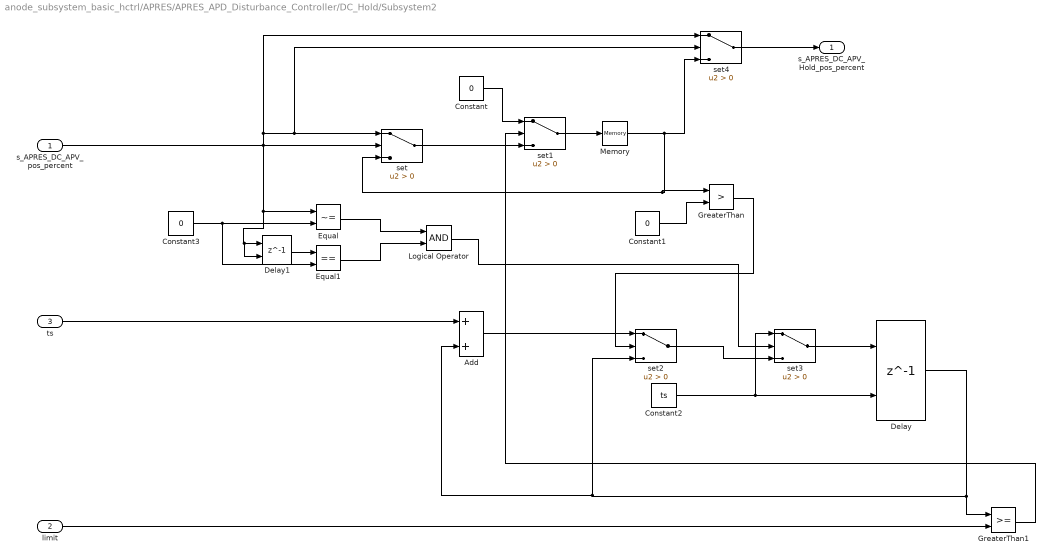
== system anode_subsystem_basic_hctrl/APRES/APRES_APD_Disturbance_Controller/DC_Hold/Subsystem2 ==
  s_APRES_DC_APV_pos_percent : Inport
  limit : Inport  Port=2
  ts : Inport  Port=3
  Add : Sum
  Constant : Constant  Value=0  OutDataTypeStr=single
  Constant1 : Constant  Value=0  OutDataTypeStr=single
  Constant2 : Constant  Value=ts  OutDataTypeStr=single
  Constant3 : Constant  Value=0  OutDataTypeStr=single
  Delay : Delay  DelayLength=1  InitialConditionSource=Input port
      settings: InputPortMap=u0,p4
  Delay1 : Delay  DelayLength=1  InitialConditionSource=Input port
      settings: InputPortMap=u0,p4
  Equal : RelationalOperator  Operator=~=  OutDataTypeStr=boolean  RndMeth=Simplest  InputSameDT=off
  Equal1 : RelationalOperator  Operator===  OutDataTypeStr=boolean  RndMeth=Simplest  InputSameDT=off
  GreaterThan : RelationalOperator  Operator=>  OutDataTypeStr=boolean  RndMeth=Simplest  InputSameDT=off
  GreaterThan1 : RelationalOperator  OutDataTypeStr=boolean  RndMeth=Simplest  InputSameDT=off
  Logical Operator : Logic  AllPortsSameDT=off  OutDataTypeStr=boolean
  Memory : Memory
  set{,1..4} (5 alike) : Switch  Criteria=u2 > Threshold  SaturateOnIntegerOverflow=off  InputSameDT=off
  s_APRES_DC_APV_Hold_pos_percent : Outport
  wires:
  set4/1 -> s_APRES_DC_APV_Hold_pos_percent/1
  set3/1 -> Delay/1
  Logical Operator/1 -> set3/2
  Equal1/1 -> Logical Operator/2
  Equal/1 -> Logical Operator/1
  Delay1/1 -> Equal1/1
  s_APRES_DC_APV_pos_percent/1 -> set/2, set/1, set4/2, set4/1, Equal/1, Delay1/1, Delay1/2
  Constant3/1 -> Equal1/2, Equal/2
  set2/1 -> set3/3
  GreaterThan/1 -> set2/2
  GreaterThan1/1 -> set1/2
  limit/1 -> GreaterThan1/2
  ts/1 -> Add/1
  Delay/1 -> Add/2, set2/3, GreaterThan1/1
  Add/1 -> set2/1
  Constant2/1 -> Delay/2, set3/1
  Constant1/1 -> GreaterThan/2
  Constant/1 -> set1/1
  set1/1 -> Memory/1
  set/1 -> set1/3
  Memory/1 -> set4/3, set/3, GreaterThan/1

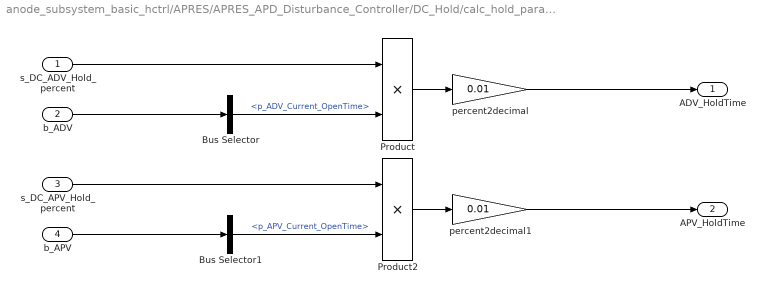
== system anode_subsystem_basic_hctrl/APRES/APRES_APD_Disturbance_Controller/DC_Hold/calc_hold_parameters ==
  s_DC_ADV_Hold_percent : Inport
  b_ADV : Inport  Port=2
  s_DC_APV_Hold_percent : Inport  Port=3
  b_APV : Inport  Port=4
  Bus Selector : BusSelector  OutputSignals=p_ADV_Current_OpenTime
  Bus Selector1 : BusSelector  OutputSignals=p_APV_Current_OpenTime
  Product : Product
  Product2 : Product
  percent2decimal : Gain  Gain=0.01
  percent2decimal1 : Gain  Gain=0.01
  ADV_HoldTime : Outport
  APV_HoldTime : Outport  Port=2
  wires:
  percent2decimal1/1 -> APV_HoldTime/1
  s_DC_APV_Hold_percent/1 -> Product2/1
  Bus Selector1/1 -> Product2/2  "<p_APV_Current_OpenTime>"
  Product/1 -> percent2decimal/1
  Bus Selector/1 -> Product/2  "<p_ADV_Current_OpenTime>"
  percent2decimal/1 -> ADV_HoldTime/1
  Product2/1 -> percent2decimal1/1
  s_DC_ADV_Hold_percent/1 -> Product/1
  b_APV/1 -> Bus Selector1/1
  b_ADV/1 -> Bus Selector/1

== matlab function anode_subsystem_basic_hctrl/APRV_VL6112 Valve_Control/Valve Lift Command Control ==
  data: m_dot input; p1 input; p2 input; T1 input; Kvs input; lift_signal output; rho_std input; W output
function [lift_signal,W]  = fcn(m_dot,p1,p2,T1,Kvs,rho_std)

% calculation based on Bürkert. Direktwirkendes 2-Wege-Standard-Proportionalventil. Datenblatt
% for calculation based on Swagelok. Valve Sizing. Technical Bulletin:
% check calculation_valve_formulas_comparison

% determine optimum valve opening based on pressure ratio for subscritical conditions
% Kvs - valve coefficient [m^3/h] at fully valve open
% lift_signal = Kv/Kvs (linear assumption)

dp = max(0,p1 - p2);            % avoid complex square root

% distinction of flow characteristics based on pressure drop
if p2/p1 > 0.5
    % low pressure drop - subsonic flow
    lift_signal = m_dot*3.6/(Kvs*514)*sqrt(T1/(p2*dp*rho_std));
    W=1;
  
else 
    % high pressure drop - sonic flow (independent of downstream pressure)
    %lift_signal = 0.05;
    lift_signal = m_dot*3.6/(Kvs*257*p1)*sqrt(T1/rho_std);
     W=2;
end
